simulink model "sistema_fisico"  (R2019a)
settings: Solver=VariableStepAuto  StartTime=0.0  StopTime=10.0  RelTol=1e-3
values from neighbouring files (symbols this model uses):
  b_cx = 1.0e6    (= 1000000)    [parametros.m]
  b_cy = 1.0e7    (= 10000000)    [parametros.m]
  b_h_eq = 2 * ( b_hd + i_h^2*b_hm ) / (r_hd^2)    (= 31004.4444444)    [parametros.m]
  b_hb = 1.0e8    (= 100000000)    [parametros.m]
  b_hEb = 2.2e9    (= 2200000000)    [parametros.m]
  b_t = 90.0    (= 90)    [parametros.m]
  b_tb = 5.0e6    (= 5000000)    [parametros.m]
  b_td_eq = ( b_td + i_t^2*b_tm ) / (r_td^2)    (= 21607.2)    [parametros.m]
  b_tw = 3.0e3    (= 3000)    [parametros.m]
  b_wu = 150    [parametros.m]
  g = Simulink.Parameter(9.80665)    [parametros.m]
  H_c = Simulink.Parameter(2.59)    [parametros.m]
  i_h = 22.0    (= 22)    [parametros.m]
  i_t = 30.0    (= 30)    [parametros.m]
  K_cy = 1.8e9    (= 1800000000)    [parametros.m]
  K_tw = 4.8e5    (= 480000)    [parametros.m]
  k_wu = 2.36e8    (= 236000000)    [parametros.m]
  l_h0 = Y_t0 - y_h0    [parametros.m]
  M_c_max = 50000    [parametros.m]
  M_c_min = 2000    [parametros.m]
  m_h_eq = 2 * ( J_hd_hEb + i_h^2*J_hm_hb ) / (r_hd^2)    (= 65137.7777778)    [parametros.m]
  M_s = 15000    [parametros.m]
  M_t = Simulink.Parameter(30000)    [parametros.m]
  m_td_eq = ( J_td + i_t^2*J_tm_tb ) / (r_td^2)    (= 30000)    [parametros.m]
  overload = false    [parametros.m]
  r_hd = 0.75    [parametros.m]
  r_td = 0.50    (= 0.5)    [parametros.m]
  T_hb_max = 5.0e4    (= 50000)    [parametros.m]
  T_hEb_max = 1.1e6    (= 1100000)    [parametros.m]
  T_tb_max = 5.0e3    (= 5000)    [parametros.m]
  v_h_max = 3.0    (= 3)    [parametros.m]
  x_l0 = x_t0    [parametros.m]
  x_t0 = W_c.Value / 2    [parametros.m]
  x_t_max_emer = x_t_max_oper.Value + 1.0    [parametros.m]
  x_t_max_oper = Simulink.Parameter(50.0)    [parametros.m]
  x_t_min_emer = x_t_min_oper.Value - 1.0    [parametros.m]
  x_t_min_oper = Simulink.Parameter(-30.0)    [parametros.m]
  x_td0 = x_t0    [parametros.m]
  y_h_max_emer = y_h_max_oper.Value + 1.0    [parametros.m]
  y_h_max_oper = Simulink.Parameter(40.0)    [parametros.m]
  y_h_min_emer = y_h_min_oper.Value - 1.0    [parametros.m]
  y_h_min_oper = Simulink.Parameter(-20.0)    [parametros.m]
  y_l0 = y_h0    [parametros.m]
  Y_t0 = 45.0    (= 45)    [parametros.m]
libraries: simulink x10
settings Model: Creator=Facundo  LastModifiedBy=Facundo

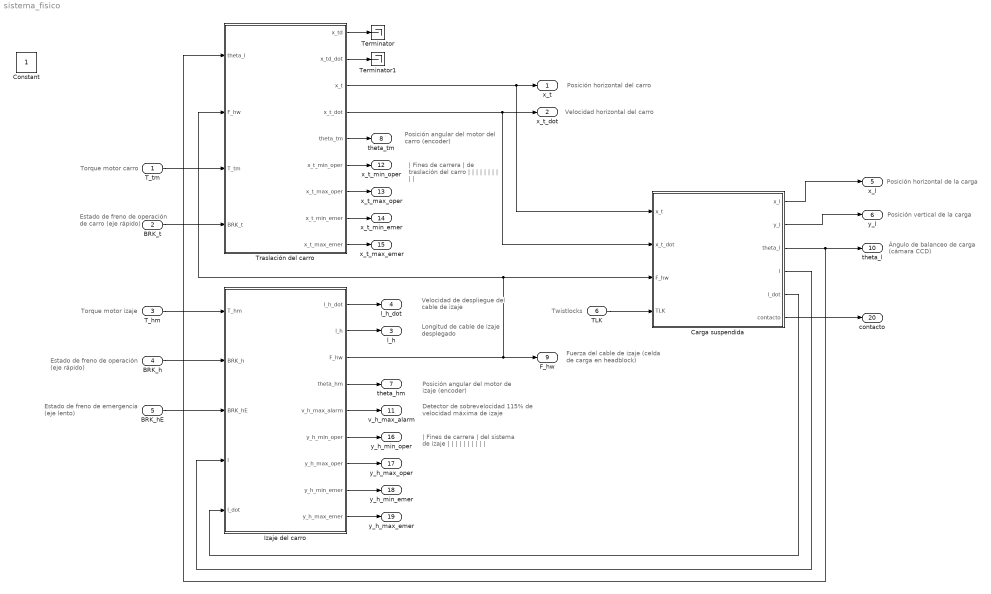
== system sistema_fisico ==
  note: Posición horizontal del carro
  note: Velocidad de despliegue
      | del cable de izaje
  note: Torque motor izaje
  note: Longitud de cable
      | de izaje desplegado
  note: Twistlocks
  note: Posición horizontal de la carga
  note: Fuerza del cable de izaje
      | (celda de carga en headblock)
  note: Detector de sobrevelocidad
      | 115% de velocidad máxima de izaje
  note: Estado de freno de emergencia
      | (eje lento)
  note: Torque motor carro
  note: Estado de freno de operación
      | (eje rápido)
  note: Posición angular del
      | motor de izaje (encoder)
  note: Posición angular del
      | motor del carro (encoder)
  note: | Fines de carrera
      | | de traslación del carro
      | |
      | |
      | |
      | |
      | |
      | |
      | |
      | |
      | |
      | |
  note: | Fines de carrera
      | | del sistema de izaje
      | |
      | |
      | |
      | |
      | |
      | |
      | |
      | |
      | |
      | |
  note: Ángulo de balanceo de carga
      | (cámara CCD)
  note: Estado de freno de
      | operación de carro
      | (eje rápido)
  note: Posición vertical de la carga
  note: Velocidad horizontal del carro
  T_tm : Inport
  BRK_t : Inport  Port=2
  T_hm : Inport  Port=3
  BRK_h : Inport  Port=4
  BRK_hE : Inport  Port=5
  TLK : Inport  Port=6  OutDataTypeStr=boolean  PortDimensions=1  SampleTime=0
  Carga suspendida : Subsystem
  Izaje del carro : Subsystem
  Terminator : Terminator
  Terminator1 : Terminator
  Traslación del carro : Subsystem
  x_t : Outport
  x_t_dot : Outport  Port=2
  l_h : Outport  Port=3
  l_h_dot : Outport  Port=4
  x_l : Outport  Port=5
  y_l : Outport  Port=6
  theta_hm : Outport  Port=7
  theta_tm : Outport  Port=8
  F_hw : Outport  Port=9
  theta_l : Outport  Port=10
  v_h_max_alarm : Outport  Port=11
  x_t_min_oper : Outport  Port=12
  x_t_max_oper : Outport  Port=13
  x_t_min_emer : Outport  Port=14
  x_t_max_emer : Outport  Port=15
  y_h_min_oper : Outport  Port=16
  y_h_max_oper : Outport  Port=17
  y_h_min_emer : Outport  Port=18
  y_h_max_emer : Outport  Port=19
  contacto : Outport  Port=20
  Constant : Constant  IOType=siggen
  wires:
  Traslación del carro/8(x_t_min_emer) -> x_t_min_emer/1
  BRK_hE/1 -> Izaje del carro/3(BRK_hE)
  Carga suspendida/2(y_l) -> y_l/1
  Izaje del carro/9(y_h_max_emer) -> y_h_max_emer/1
  Carga suspendida/3(theta_l) -> theta_l/1, Traslación del carro/1(theta_l)
  T_hm/1 -> Izaje del carro/1(T_hm)
  Izaje del carro/6(y_h_min_oper) -> y_h_min_oper/1
  Carga suspendida/1(x_l) -> x_l/1
  Izaje del carro/5(v_h_max_alarm) -> v_h_max_alarm/1
  T_tm/1 -> Traslación del carro/3(T_tm)
  Traslación del carro/4(x_t_dot) -> Carga suspendida/2(x_t_dot), x_t_dot/1
  Izaje del carro/4(theta_hm) -> theta_hm/1
  Traslación del carro/2(x_td_dot) -> Terminator1/1
  Carga suspendida/5(l_dot) -> Izaje del carro/5(l_dot)
  Izaje del carro/1(l_h_dot) -> l_h_dot/1
  Traslación del carro/5(theta_tm) -> theta_tm/1
  Izaje del carro/7(y_h_max_oper) -> y_h_max_oper/1
  Izaje del carro/2(l_h) -> l_h/1
  Izaje del carro/3(F_hw) -> F_hw/1, Carga suspendida/3(F_hw), Traslación del carro/2(F_hw)
  TLK/1 -> Carga suspendida/4(TLK)
  Traslación del carro/9(x_t_max_emer) -> x_t_max_emer/1
  Traslación del carro/1(x_td) -> Terminator/1
  Carga suspendida/6(contacto) -> contacto/1
  BRK_t/1 -> Traslación del carro/4(BRK_t)
  Traslación del carro/3(x_t) -> Carga suspendida/1(x_t), x_t/1
  Traslación del carro/6(x_t_min_oper) -> x_t_min_oper/1
  BRK_h/1 -> Izaje del carro/2(BRK_h)
  Traslación del carro/7(x_t_max_oper) -> x_t_max_oper/1
  Izaje del carro/8(y_h_min_emer) -> y_h_min_emer/1
  Carga suspendida/4(l) -> Izaje del carro/4(l)

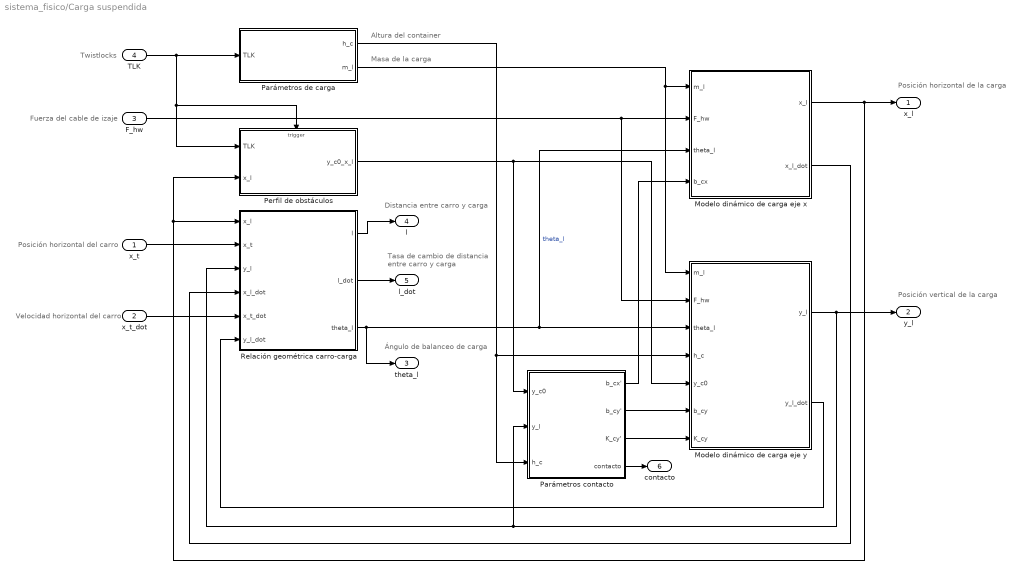
== system sistema_fisico/Carga suspendida ==
  note: Twistlocks
  note: Altura del container
  note: Posición horizontal del carro
  note: Posición vertical de la carga
  note: Velocidad horizontal del carro
  note: Distancia entre carro y carga
  note: Fuerza del cable de izaje
  note: Ángulo de balanceo de carga
  note: Tasa de cambio de distancia
      | entre carro y carga
  note: Masa de la carga
  note: Posición horizontal de la carga
  x_t : Inport  OutDataTypeStr=double  PortDimensions=1  SampleTime=0
  x_t_dot : Inport  Port=2  OutDataTypeStr=double  PortDimensions=1  SampleTime=0
  F_hw : Inport  Port=3  OutDataTypeStr=double  PortDimensions=1  SampleTime=0
  TLK : Inport  Port=4  OutDataTypeStr=boolean  PortDimensions=1  SampleTime=0
  Modelo dinámico de carga eje x : Subsystem
  Modelo dinámico de carga eje y : Subsystem
  Parámetros contacto : Subsystem
  Parámetros de carga : Subsystem
  Perfil de obstáculos : Subsystem
  Relación geométrica carro-carga : Subsystem
  x_l : Outport  OutDataTypeStr=double  PortDimensions=1  SampleTime=0
  y_l : Outport  Port=2  OutDataTypeStr=double  PortDimensions=1  SampleTime=0
  theta_l : Outport  Port=3  OutDataTypeStr=double  PortDimensions=1  SampleTime=0
  l : Outport  Port=4  OutDataTypeStr=double  PortDimensions=1  SampleTime=0
  l_dot : Outport  Port=5  OutDataTypeStr=double  PortDimensions=1  SampleTime=0
  contacto : Outport  Port=6  OutDataTypeStr=boolean  PortDimensions=1  SampleTime=0
  wires:
  Parámetros de carga/2(m_l) -> Modelo dinámico de carga eje y/1(m_l), Modelo dinámico de carga eje x/1(m_l)
  F_hw/1 -> Modelo dinámico de carga eje y/2(F_hw), Modelo dinámico de carga eje x/2(F_hw)
  Relación geométrica carro-carga/2(l_dot) -> l_dot/1
  x_t_dot/1 -> Relación geométrica carro-carga/5(x_t_dot)
  Modelo dinámico de carga eje y/1(y_l) -> y_l/1, Parámetros contacto/2(y_l), Relación geométrica carro-carga/3(y_l)
  Modelo dinámico de carga eje x/2(x_l_dot) -> Relación geométrica carro-carga/4(x_l_dot)
  Modelo dinámico de carga eje y/2(y_l_dot) -> Relación geométrica carro-carga/6(y_l_dot)
  x_t/1 -> Relación geométrica carro-carga/2(x_t)
  Modelo dinámico de carga eje x/1(x_l) -> Perfil de obstáculos/2(x_l), Relación geométrica carro-carga/1(x_l), x_l/1
  Relación geométrica carro-carga/3(theta_l) -> theta_l/1, Modelo dinámico de carga eje x/3(theta_l), Modelo dinámico de carga eje y/3(theta_l)  "theta_l"
  Parámetros contacto/1(b_cx') -> Modelo dinámico de carga eje x/4(b_cx)
  Parámetros contacto/2(b_cy') -> Modelo dinámico de carga eje y/6(b_cy)
  Parámetros contacto/3(K_cy') -> Modelo dinámico de carga eje y/7(K_cy)
  Relación geométrica carro-carga/1(l) -> l/1
  Parámetros contacto/4(contacto) -> contacto/1
  Parámetros de carga/1(h_c) -> Modelo dinámico de carga eje y/4(h_c), Parámetros contacto/3(h_c)
  Perfil de obstáculos/1(y_c0_x_l) -> Parámetros contacto/1(y_c0), Modelo dinámico de carga eje y/5(y_c0)
  TLK/1 -> Parámetros de carga/1(TLK), Perfil de obstáculos/Trigger, Perfil de obstáculos/1(TLK)

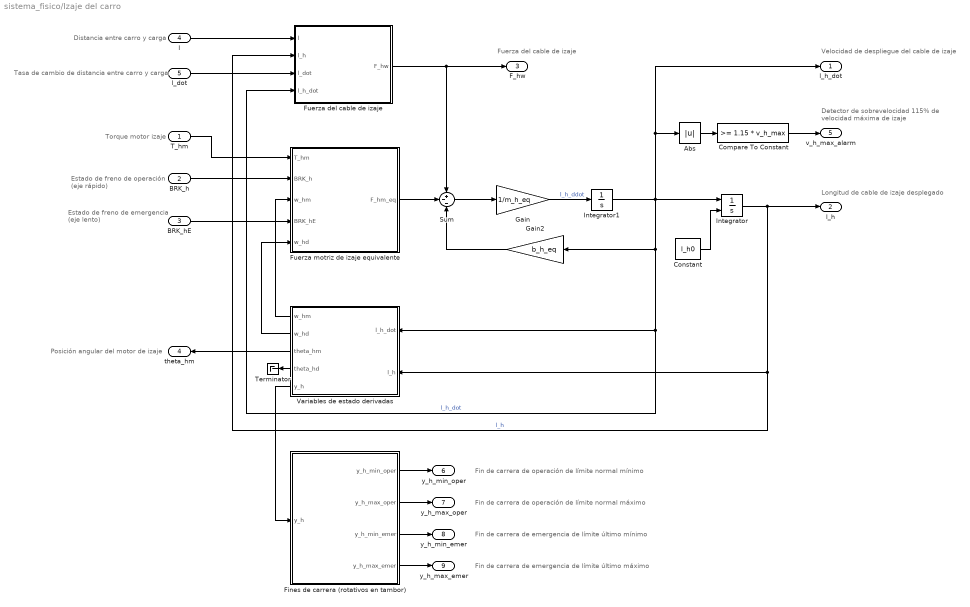
== system sistema_fisico/Izaje del carro ==
  note: Detector de sobrevelocidad
      | 115% de velocidad máxima de izaje
  note: Posición angular del motor de izaje
  note: Longitud de cable de izaje desplegado
  note: Velocidad de despliegue del cable de izaje
  note: Torque motor izaje
  note: Estado de freno de emergencia
      | (eje lento)
  note: Tasa de cambio de distancia entre carro y carga
  note: Estado de freno de operación
      | (eje rápido)
  note: Distancia entre carro y carga
  note: Fuerza del cable de izaje
  note: Fin de carrera de operación de límite normal mínimo
  note: Fin de carrera de emergencia de límite último máximo
  note: Fin de carrera de emergencia de límite último mínimo
  note: Fin de carrera de operación de límite normal máximo
  T_hm : Inport
  BRK_h : Inport  Port=2
  BRK_hE : Inport  Port=3
  l : Inport  Port=4
  l_dot : Inport  Port=5
  Abs : Abs
  Compare To Constant : simulink/Logic and Bit Operations/Compare To Constant  relop=>=  const=1.15 * v_h_max  OutDataTypeStr=boolean
  Constant : Constant  Value=l_h0
  Fines de carrera (rotativos en tambor) : Subsystem
  Fuerza del cable de izaje : Subsystem
  Fuerza motriz de izaje equivalente : Subsystem
  Gain : Gain  Gain=1/m_h_eq
  Gain2 : Gain  Gain=b_h_eq
  Integrator : Integrator  InitialConditionSource=external
  Integrator1 : Integrator
  Sum : Sum  Inputs=+--
  Terminator : Terminator
  Variables de estado derivadas : Subsystem
  l_h_dot : Outport
  l_h : Outport  Port=2
  F_hw : Outport  Port=3
  theta_hm : Outport  Port=4
  v_h_max_alarm : Outport  Port=5
  y_h_min_oper : Outport  Port=6  OutDataTypeStr=boolean  PortDimensions=1  SampleTime=0
  y_h_max_oper : Outport  Port=7  OutDataTypeStr=boolean  PortDimensions=1  SampleTime=0
  y_h_min_emer : Outport  Port=8  OutDataTypeStr=boolean  PortDimensions=1  SampleTime=0
  y_h_max_emer : Outport  Port=9  OutDataTypeStr=boolean  PortDimensions=1  SampleTime=0
  wires:
  Integrator/1 -> l_h/1, Fuerza del cable de izaje/2(l_h), Variables de estado derivadas/2(l_h)  "l_h"
  Integrator1/1 -> l_h_dot/1, Abs/1, Fuerza del cable de izaje/4(l_h_dot), Variables de estado derivadas/1(l_h_dot), Gain2/1, Integrator/1  "l_h_dot"
  T_hm/1 -> Fuerza motriz de izaje equivalente/1(T_hm)
  l/1 -> Fuerza del cable de izaje/1(l)
  l_dot/1 -> Fuerza del cable de izaje/3(l_dot)
  Fuerza del cable de izaje/1(F_hw) -> F_hw/1, Sum/1
  Gain2/1 -> Sum/3
  Fuerza motriz de izaje equivalente/1(F_hm_eq) -> Sum/2
  Variables de estado derivadas/1(w_hm) -> Fuerza motriz de izaje equivalente/3(w_hm)
  Sum/1 -> Gain/1
  Variables de estado derivadas/2(w_hd) -> Fuerza motriz de izaje equivalente/5(w_hd)
  BRK_h/1 -> Fuerza motriz de izaje equivalente/2(BRK_h)
  BRK_hE/1 -> Fuerza motriz de izaje equivalente/4(BRK_hE)
  Gain/1 -> Integrator1/1  "l_h_ddot"
  Constant/1 -> Integrator/2
  Variables de estado derivadas/3(theta_hm) -> theta_hm/1
  Abs/1 -> Compare To Constant/1
  Compare To Constant/1 -> v_h_max_alarm/1
  Fines de carrera (rotativos en tambor)/1(y_h_min_oper) -> y_h_min_oper/1
  Fines de carrera (rotativos en tambor)/4(y_h_max_emer) -> y_h_max_emer/1
  Fines de carrera (rotativos en tambor)/3(y_h_min_emer) -> y_h_min_emer/1
  Fines de carrera (rotativos en tambor)/2(y_h_max_oper) -> y_h_max_oper/1
  Variables de estado derivadas/5(y_h) -> Fines de carrera (rotativos en tambor)/1(y_h)
  Variables de estado derivadas/4(theta_hd) -> Terminator/1

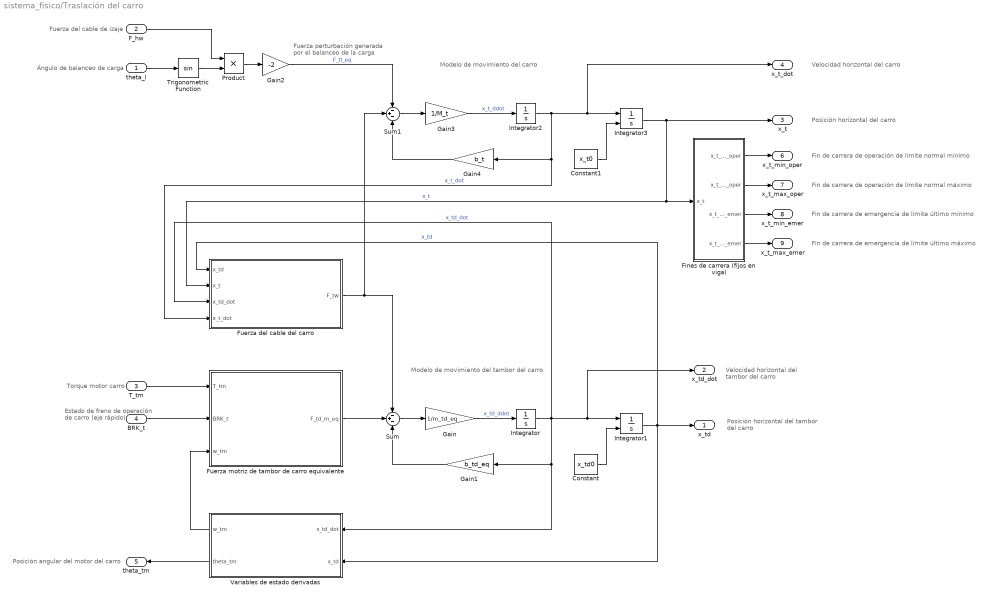
== system sistema_fisico/Traslación del carro ==
  note: Posición angular del motor del carro
  note: Velocidad horizontal
      | del tambor del carro
  note: Modelo de movimiento del tambor del carro
  note: Modelo de movimiento del carro
  note: Velocidad horizontal del carro
  note: Estado de freno de
      | operación de carro
      | (eje rápido)
  note: Fuerza del cable de izaje
  note: Fuerza perturbación generada
      | por el balanceo de la carga
  note: Posición horizontal del carro
  note: Torque motor carro
  note: Ángulo de balanceo de carga
  note: Posición horizontal
      | del tambor del carro
  note: Fin de carrera de operación de límite normal mínimo
  note: Fin de carrera de operación de límite normal máximo
  note: Fin de carrera de emergencia de límite último mínimo
  note: Fin de carrera de emergencia de límite último máximo
  theta_l : Inport  OutDataTypeStr=double  PortDimensions=1  SampleTime=0
  F_hw : Inport  Port=2  OutDataTypeStr=double  PortDimensions=1  SampleTime=0
  T_tm : Inport  Port=3
  BRK_t : Inport  Port=4
  Constant : Constant  Value=x_td0
  Constant1 : Constant  Value=x_t0
  Fines de carrera (fijos en viga) : Subsystem
  Fuerza del cable del carro : Subsystem
  Fuerza motriz de tambor de carro equivalente : Subsystem
  Gain : Gain  Gain=1/m_td_eq
  Gain1 : Gain  Gain=b_td_eq
  Gain2 : Gain  Gain=-2
  Gain3 : Gain  Gain=1/M_t
  Gain4 : Gain  Gain=b_t
  Integrator : Integrator
  Integrator1 : Integrator  InitialConditionSource=external
  Integrator2 : Integrator
  Integrator3 : Integrator  InitialConditionSource=external
  Product : Product
  Sum : Sum  Inputs=-+-
  Sum1 : Sum  Inputs=-+-
  Trigonometric Function : Trigonometry
  Variables de estado derivadas : Subsystem
  x_td : Outport  OutDataTypeStr=double  PortDimensions=1  SampleTime=0
  x_td_dot : Outport  Port=2  OutDataTypeStr=double  PortDimensions=1  SampleTime=0
  x_t : Outport  Port=3  OutDataTypeStr=double  PortDimensions=1  SampleTime=0
  x_t_dot : Outport  Port=4  OutDataTypeStr=double  PortDimensions=1  SampleTime=0
  theta_tm : Outport  Port=5  OutDataTypeStr=double  PortDimensions=1  SampleTime=0
  x_t_min_oper : Outport  Port=6  OutDataTypeStr=boolean  PortDimensions=1  SampleTime=0
  x_t_max_oper : Outport  Port=7  OutDataTypeStr=boolean  PortDimensions=1  SampleTime=0
  x_t_min_emer : Outport  Port=8  OutDataTypeStr=boolean  PortDimensions=1  SampleTime=0
  x_t_max_emer : Outport  Port=9  OutDataTypeStr=boolean  PortDimensions=1  SampleTime=0
  wires:
  Integrator1/1 -> Variables de estado derivadas/2(x_td), Fuerza del cable del carro/1(x_td), x_td/1  "x_td"
  Gain3/1 -> Integrator2/1  "x_t_ddot"
  Fuerza del cable del carro/1(F_tw) -> Sum1/2, Sum/1
  Sum/1 -> Gain/1
  Integrator/1 -> Fuerza del cable del carro/3(x_td_dot), Variables de estado derivadas/1(x_td_dot), Gain1/1, x_td_dot/1, Integrator1/1  "x_td_dot"
  F_hw/1 -> Product/1
  Fuerza motriz de tambor de carro equivalente/1(F_td_m_eq) -> Sum/2
  Constant/1 -> Integrator1/2
  Gain1/1 -> Sum/3
  Integrator2/1 -> Fuerza del cable del carro/4(x_t_dot), Gain4/1, x_t_dot/1, Integrator3/1  "x_t_dot"
  Sum1/1 -> Gain3/1
  theta_l/1 -> Trigonometric Function/1
  Gain4/1 -> Sum1/3
  Integrator3/1 -> x_t/1, Fuerza del cable del carro/2(x_t), Fines de carrera (fijos en viga)/1(x_t)  "x_t"
  Gain2/1 -> Sum1/1  "F_tl_eq"
  T_tm/1 -> Fuerza motriz de tambor de carro equivalente/1(T_tm)
  BRK_t/1 -> Fuerza motriz de tambor de carro equivalente/2(BRK_t)
  Variables de estado derivadas/1(w_tm) -> Fuerza motriz de tambor de carro equivalente/3(w_tm)
  Constant1/1 -> Integrator3/2
  Trigonometric Function/1 -> Product/2
  Product/1 -> Gain2/1
  Gain/1 -> Integrator/1  "x_td_ddot"
  Variables de estado derivadas/2(theta_tm) -> theta_tm/1
  Fines de carrera (fijos en viga)/1(x_t_min_oper) -> x_t_min_oper/1
  Fines de carrera (fijos en viga)/2(x_t_max_oper) -> x_t_max_oper/1
  Fines de carrera (fijos en viga)/3(x_t_min_emer) -> x_t_min_emer/1
  Fines de carrera (fijos en viga)/4(x_t_max_emer) -> x_t_max_emer/1

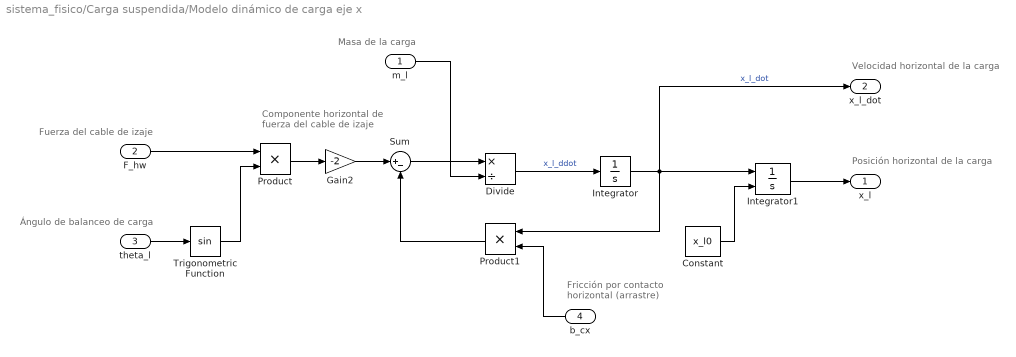
== system sistema_fisico/Carga suspendida/Modelo dinámico de carga eje x ==
  note: Componente horizontal de
      | fuerza del cable de izaje
  note: Posición horizontal de la carga
  note: Velocidad horizontal de la carga
  note: Fuerza del cable de izaje
  note: Masa de la carga
  note: Fricción por contacto
      | horizontal (arrastre)
  note: Ángulo de balanceo de carga
  m_l : Inport  OutDataTypeStr=double  PortDimensions=1  SampleTime=0
  F_hw : Inport  Port=2  OutDataTypeStr=double  PortDimensions=1  SampleTime=0
  theta_l : Inport  Port=3  OutDataTypeStr=double  PortDimensions=1  SampleTime=0
  b_cx : Inport  Port=4  OutDataTypeStr=double  PortDimensions=1  SampleTime=0
  Constant : Constant  Value=x_l0
  Divide : Product  Inputs=*/
  Gain2 : Gain  Gain=-2
  Integrator : Integrator
  Integrator1 : Integrator  InitialConditionSource=external
  Product : Product
  Product1 : Product
  Sum : Sum  Inputs=|+-
  Trigonometric Function : Trigonometry
  x_l : Outport  OutDataTypeStr=double  PortDimensions=1  SampleTime=0
  x_l_dot : Outport  Port=2  OutDataTypeStr=double  PortDimensions=1  SampleTime=0
  wires:
  F_hw/1 -> Product/1
  Product1/1 -> Sum/2
  theta_l/1 -> Trigonometric Function/1
  b_cx/1 -> Product1/2
  Sum/1 -> Divide/1
  Integrator/1 -> x_l_dot/1, Integrator1/1, Product1/1  "x_l_dot"
  Product/1 -> Gain2/1
  Divide/1 -> Integrator/1  "x_l_ddot"
  Constant/1 -> Integrator1/2
  Integrator1/1 -> x_l/1
  Gain2/1 -> Sum/1
  m_l/1 -> Divide/2
  Trigonometric Function/1 -> Product/2

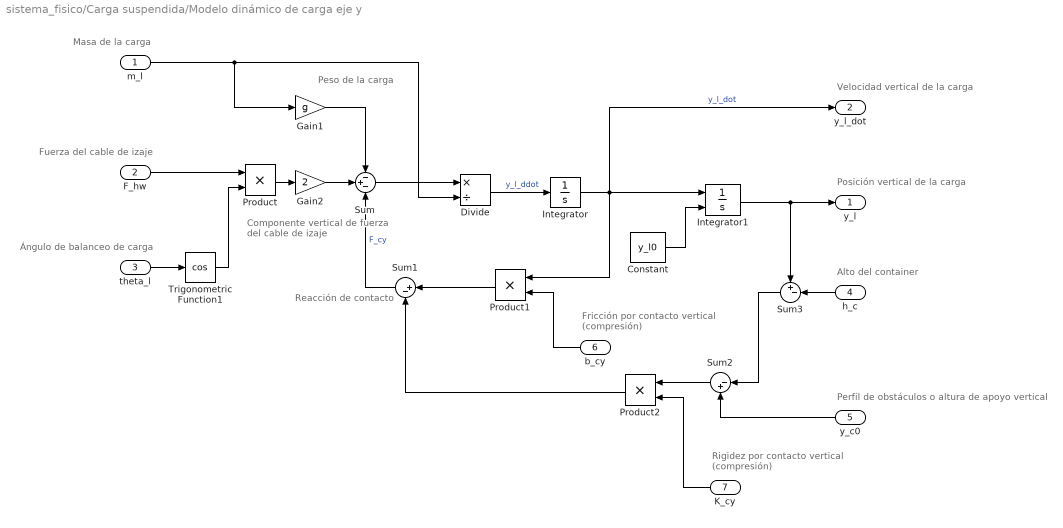
== system sistema_fisico/Carga suspendida/Modelo dinámico de carga eje y ==
  note: Reacción de contacto
  note: Peso de la carga
  note: Componente vertical de
      | fuerza del cable de izaje
  note: Posición vertical de la carga
  note: Velocidad vertical de la carga
  note: Fricción por contacto
      | vertical (compresión)
  note: Rigidez por contacto
      | vertical (compresión)
  note: Masa de la carga
  note: Fuerza del cable de izaje
  note: Perfil de obstáculos o altura de apoyo vertical
  note: Alto del container
  note: Ángulo de balanceo de carga
  m_l : Inport  OutDataTypeStr=double  PortDimensions=1  SampleTime=0
  F_hw : Inport  Port=2  OutDataTypeStr=double  PortDimensions=1  SampleTime=0
  theta_l : Inport  Port=3  OutDataTypeStr=double  PortDimensions=1  SampleTime=0
  h_c : Inport  Port=4  OutDataTypeStr=double  PortDimensions=1  SampleTime=0
  y_c0 : Inport  Port=5  OutDataTypeStr=double  PortDimensions=1  SampleTime=0
  b_cy : Inport  Port=6  OutDataTypeStr=double  PortDimensions=1  SampleTime=0
  K_cy : Inport  Port=7  OutDataTypeStr=double  PortDimensions=1  SampleTime=0
  Constant : Constant  Value=y_l0
  Divide : Product  Inputs=*/
  Gain1 : Gain  Gain=g
  Gain2 : Gain  Gain=2
  Integrator : Integrator
  Integrator1 : Integrator  InitialConditionSource=external
  Product : Product
  Product1 : Product
  Product2 : Product
  Sum : Sum  Inputs=-+-
  Sum1 : Sum  Inputs=|+-
  Sum2 : Sum  Inputs=|-+
  Sum3 : Sum  Inputs=+-|
  Trigonometric Function1 : Trigonometry  Operator=cos
  y_l : Outport  OutDataTypeStr=double  PortDimensions=1  SampleTime=0
  y_l_dot : Outport  Port=2  OutDataTypeStr=double  PortDimensions=1  SampleTime=0
  wires:
  F_hw/1 -> Product/1
  theta_l/1 -> Trigonometric Function1/1
  b_cy/1 -> Product1/2
  Integrator/1 -> y_l_dot/1, Integrator1/1, Product1/1  "y_l_dot"
  Divide/1 -> Integrator/1  "y_l_ddot"
  Constant/1 -> Integrator1/2
  Integrator1/1 -> y_l/1, Sum3/1
  Product/1 -> Gain2/1
  Product1/1 -> Sum1/1
  Sum1/1 -> Sum/3  "F_cy"
  Gain1/1 -> Sum/1
  y_c0/1 -> Sum2/2
  Sum2/1 -> Product2/1
  K_cy/1 -> Product2/2
  Product2/1 -> Sum1/2
  Gain2/1 -> Sum/2
  Sum/1 -> Divide/1
  m_l/1 -> Gain1/1, Divide/2
  h_c/1 -> Sum3/2
  Sum3/1 -> Sum2/1
  Trigonometric Function1/1 -> Product/2

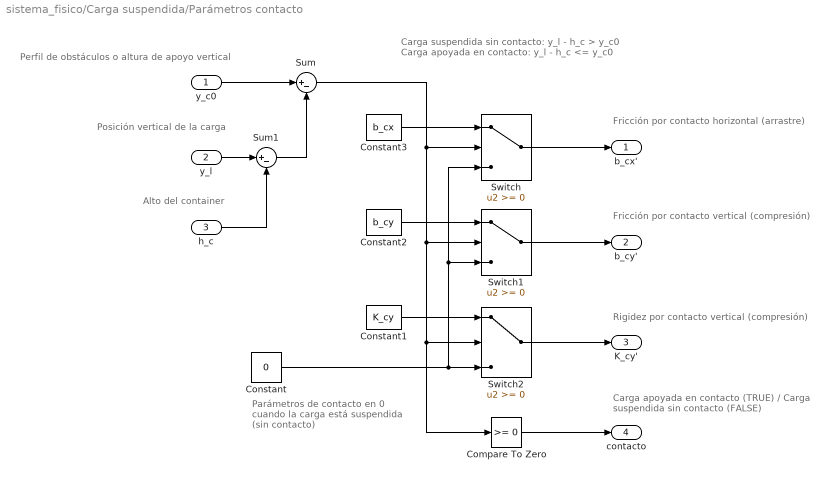
== system sistema_fisico/Carga suspendida/Parámetros contacto ==
  note: Fricción por contacto horizontal (arrastre)
  note: Fricción por contacto vertical (compresión)
  note: Rigidez por contacto vertical (compresión)
  note: Perfil de obstáculos o altura de apoyo vertical
  note: Posición vertical de la carga
  note: Alto del container
  note: Parámetros de contacto en 0
      | cuando la carga está suspendida
      | (sin contacto)
  note: Carga suspendida sin contacto: y_l - h_c > y_c0
      | Carga apoyada en contacto: y_l - h_c <= y_c0
  note: Carga apoyada en contacto (TRUE) /
      | Carga suspendida sin contacto (FALSE)
  y_c0 : Inport  OutDataTypeStr=double  PortDimensions=1  SampleTime=0
  y_l : Inport  Port=2  OutDataTypeStr=double  PortDimensions=1  SampleTime=0
  h_c : Inport  Port=3  OutDataTypeStr=double  PortDimensions=1  SampleTime=0
  Compare To Zero : simulink/Logic and Bit Operations/Compare To Zero  relop=>=  OutDataTypeStr=boolean
  Constant : Constant  Value=0
  Constant1 : Constant  Value=K_cy
  Constant2 : Constant  Value=b_cy
  Constant3 : Constant  Value=b_cx
  Sum : Sum  Inputs=|+-
  Sum1 : Sum  Inputs=|+-
  Switch : Switch
  Switch1 : Switch
  Switch2 : Switch
  b_cx' : Outport  OutDataTypeStr=double  PortDimensions=1  SampleTime=0
  b_cy' : Outport  Port=2  OutDataTypeStr=double  PortDimensions=1  SampleTime=0
  K_cy' : Outport  Port=3  OutDataTypeStr=double  PortDimensions=1  SampleTime=0
  contacto : Outport  Port=4  OutDataTypeStr=boolean  PortDimensions=1  SampleTime=0
  wires:
  y_c0/1 -> Sum/1
  Constant2/1 -> Switch1/1
  Constant1/1 -> Switch2/1
  Switch/1 -> b_cx'/1
  Sum/1 -> Switch1/2, Compare To Zero/1, Switch2/2, Switch/2
  Switch2/1 -> K_cy'/1
  Switch1/1 -> b_cy'/1
  Constant/1 -> Switch/3, Switch1/3, Switch2/3
  Constant3/1 -> Switch/1
  Sum1/1 -> Sum/2
  y_l/1 -> Sum1/1
  h_c/1 -> Sum1/2
  Compare To Zero/1 -> contacto/1

== system sistema_fisico/Carga suspendida/Parámetros de carga ==
  note: Twistlocks
  note: Masa de la carga total
  note: Alto del container
      | (afecta altura inferior)
  note: Masa del spreader
  note: Masa del contenedor
      | y carga
  TLK : Inport  OutDataTypeStr=boolean  PortDimensions=1  SampleTime=0
  "Generate random load " : Subsystem  TreatAsAtomicUnit=on
  Sum : Sum  Inputs=++|
  Switch : Switch  Criteria=u2 ~= 0
  Switch1 : Switch  Criteria=u2 ~= 0
  h_c1 : Constant  Value=H_c
  h_c2 : Constant  Value=0
  h_c3 : Constant  Value=M_s
  h_c4 : Constant  Value=0
  h_c : Outport
  m_l : Outport  Port=2
  wires:
  TLK/1 -> "Generate random load "/Trigger, Switch1/2, Switch/2
  Switch/1 -> h_c/1
  Sum/1 -> m_l/1
  Switch1/1 -> Sum/2  "M_cx"
  "Generate random load "/1(M_cx) -> Switch1/1
  h_c3/1 -> Sum/1  "M_s"
  h_c2/1 -> Switch/3
  h_c4/1 -> Switch1/3
  h_c1/1 -> Switch/1

== system sistema_fisico/Carga suspendida/Perfil de obstáculos ==
  note: Perfil de obstáculos para x_l
  note: Se actualiza el perfil de obstá culos cuando
      | se cierran (TLK ↑) o abren (TLK ↓) los twistlocks
  note: Perfil de obstáculos
  note: Guarda perfil de obstáculos en workspace
      | para posterior análisis (plot_perfil_obstaculos.m)
  TLK : Inport  PortDimensions=1
  x_l : Inport  Port=2  OutDataTypeStr=double  PortDimensions=1
  Trigger : TriggerPort  TriggerType=either  VariantControl=Variant  PortDimensions=1
  Constant : Constant  Value=H_c
  Constant1 : Constant  Value=x_t_min_oper
  Constant2 : Constant  Value=x_t_max_oper
  Constant3 : Constant  Value=y_h_min_oper
  MATLAB Function : MATLAB Function  TreatAsAtomicUnit=on
  To Workspace : ToWorkspace  VariableName=y_c0  SaveFormat=Structure With Time  SampleTime=-1
  y_c0_x_l : Outport  OutDataTypeStr=double  PortDimensions=1  InitialOutput=y_h_min_oper
  wires:
  MATLAB Function/1(y_c0_x_l) -> y_c0_x_l/1
  TLK/1 -> MATLAB Function/2(TLK)
  x_l/1 -> MATLAB Function/1(x_l)
  Constant/1 -> MATLAB Function/3(H_c)
  Constant1/1 -> MATLAB Function/4(x_t_min_oper)
  Constant2/1 -> MATLAB Function/5(x_t_max_oper)
  Constant3/1 -> MATLAB Function/6(y_h_min_oper)
  MATLAB Function/2(y_c0) -> To Workspace/1

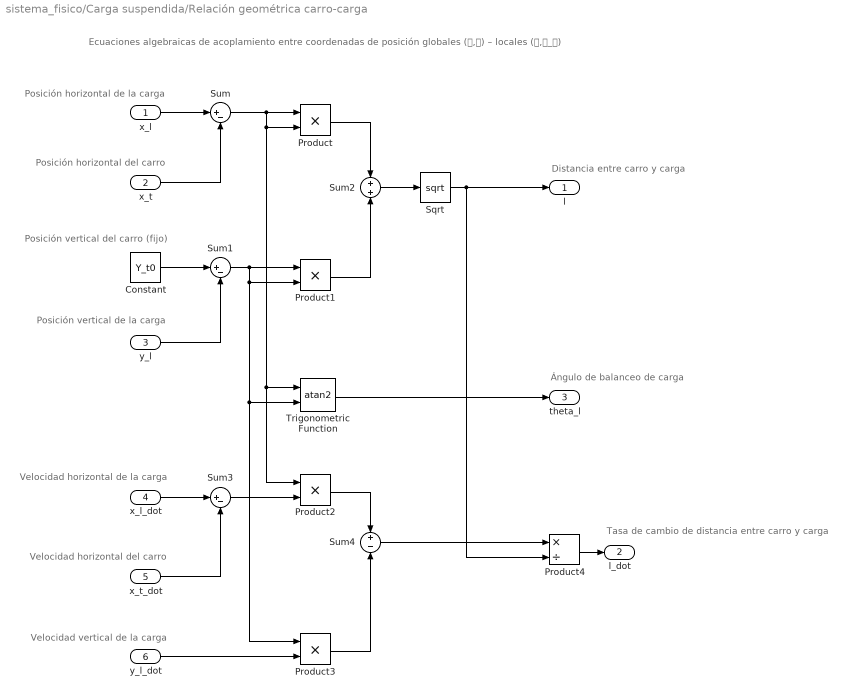
== system sistema_fisico/Carga suspendida/Relación geométrica carro-carga ==
  note: Ecuaciones algebraicas de acoplamiento entre coordenadas de posición globales (𝑥,𝑦) – locales (𝑙,𝜃_𝑙)
  note: Posición horizontal de la carga
  note: Posición horizontal del carro
  note: Posición vertical del carro (fijo)
  note: Posición vertical de la carga
  note: Distancia entre carro y carga
  note: Tasa de cambio de distancia entre carro y carga
  note: Ángulo de balanceo de carga
  note: Velocidad horizontal de la carga
  note: Velocidad horizontal del carro
  note: Velocidad vertical de la carga
  x_l : Inport
  x_t : Inport  Port=2
  y_l : Inport  Port=3
  x_l_dot : Inport  Port=4
  x_t_dot : Inport  Port=5
  y_l_dot : Inport  Port=6
  Constant : Constant  Value=Y_t0
  Product{,1..3} (4 alike) : Product
  Product4 : Product  Inputs=*/
  Sqrt : Sqrt  SaturateOnIntegerOverflow=on
  Sum : Sum  Inputs=|+-
  Sum1 : Sum  Inputs=|+-
  Sum2 : Sum  Inputs=+|+
  Sum3 : Sum  Inputs=|+-
  Sum4 : Sum  Inputs=+|-
  Trigonometric Function : Trigonometry  Operator=atan2
  l : Outport
  l_dot : Outport  Port=2
  theta_l : Outport  Port=3
  wires:
  x_t/1 -> Sum/2
  x_l/1 -> Sum/1
  Sum/1 -> Product/1, Product2/1, Trigonometric Function/1, Product/2
  Product/1 -> Sum2/1
  y_l/1 -> Sum1/2
  Sum1/1 -> Product1/1, Product3/1, Trigonometric Function/2, Product1/2
  Constant/1 -> Sum1/1
  Product1/1 -> Sum2/2
  Sum2/1 -> Sqrt/1
  Trigonometric Function/1 -> theta_l/1
  x_l_dot/1 -> Sum3/1
  x_t_dot/1 -> Sum3/2
  Sum3/1 -> Product2/2
  y_l_dot/1 -> Product3/2
  Product2/1 -> Sum4/1
  Product3/1 -> Sum4/2
  Sum4/1 -> Product4/1
  Product4/1 -> l_dot/1
  Sqrt/1 -> Product4/2, l/1

== system sistema_fisico/Izaje del carro/Fines de carrera (rotativos en tambor) ==
  note: Fines de carrera son rotativos sobre tambor (theta_hd). Por simplicidad se usa la variable equivalente lineal (y_h)
  note: Fin de carrera de operación de límite normal mínimo
  note: Fin de carrera de operación de límite normal máximo
  note: Fin de carrera de emergencia de límite último mínimo
  note: Fin de carrera de operación de límite último máximo
  note: Altura de la carga sin balanceo
  y_h : Inport
  Compare To Constant : simulink/Logic and Bit Operations/Compare To Constant  relop=<=  const=y_h_min_oper  OutDataTypeStr=boolean
  Compare To Constant1 : simulink/Logic and Bit Operations/Compare To Constant  relop=>=  const=y_h_max_oper  OutDataTypeStr=boolean
  Compare To Constant2 : simulink/Logic and Bit Operations/Compare To Constant  relop=<=  const=y_h_min_emer  OutDataTypeStr=boolean
  Compare To Constant3 : simulink/Logic and Bit Operations/Compare To Constant  relop=>=  const=y_h_max_emer  OutDataTypeStr=boolean
  y_h_min_oper : Outport  OutDataTypeStr=boolean  PortDimensions=1  SampleTime=0
  y_h_max_oper : Outport  Port=2  OutDataTypeStr=boolean  PortDimensions=1  SampleTime=0
  y_h_min_emer : Outport  Port=3  OutDataTypeStr=boolean  PortDimensions=1  SampleTime=0
  y_h_max_emer : Outport  Port=4  OutDataTypeStr=boolean  PortDimensions=1  SampleTime=0
  wires:
  Compare To Constant2/1 -> y_h_min_emer/1
  Compare To Constant/1 -> y_h_min_oper/1
  Compare To Constant1/1 -> y_h_max_oper/1
  y_h/1 -> Compare To Constant3/1, Compare To Constant2/1, Compare To Constant1/1, Compare To Constant/1
  Compare To Constant3/1 -> y_h_max_emer/1

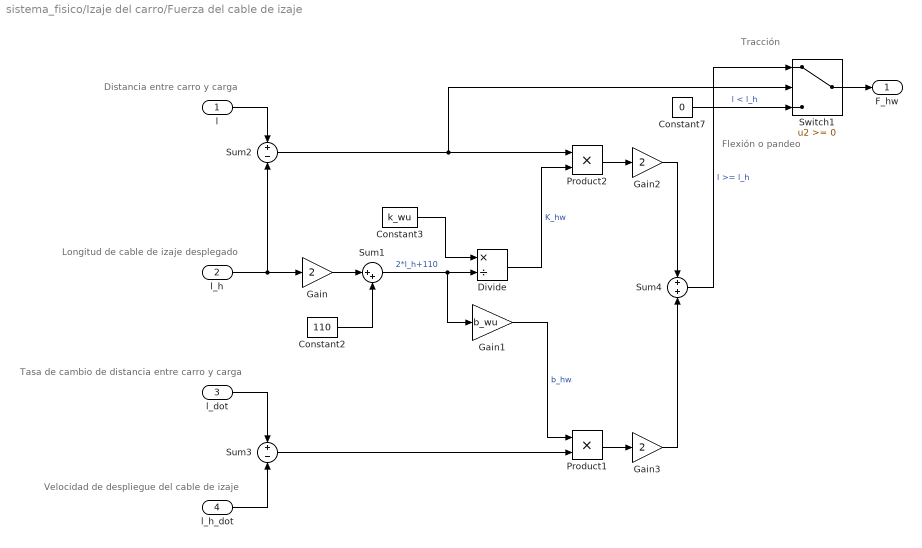
== system sistema_fisico/Izaje del carro/Fuerza del cable de izaje ==
  note: Flexión o pandeo
  note: Tracción
  note: Distancia entre carro y carga
  note: Tasa de cambio de distancia entre carro y carga
  note: Longitud de cable de izaje desplegado
  note: Velocidad de despliegue del cable de izaje
  l : Inport
  l_h : Inport  Port=2
  l_dot : Inport  Port=3
  l_h_dot : Inport  Port=4
  Constant2 : Constant  Value=110
  Constant3 : Constant  Value=k_wu
  Constant7 : Constant  Value=0
  Divide : Product  Inputs=*/
  Gain : Gain  Gain=2
  Gain1 : Gain  Gain=b_wu
  Gain2 : Gain  Gain=2
  Gain3 : Gain  Gain=2
  Product1 : Product
  Product2 : Product
  Sum1 : Sum  Inputs=|++
  Sum2 : Sum  Inputs=+-
  Sum3 : Sum  Inputs=+-
  Sum4 : Sum
  Switch1 : Switch
  F_hw : Outport
  wires:
  l_dot/1 -> Sum3/1
  Constant2/1 -> Sum1/2
  Sum1/1 -> Gain1/1, Divide/2  "2*l_h+110"
  l/1 -> Sum2/1
  Product1/1 -> Gain3/1
  Sum3/1 -> Product1/2
  l_h_dot/1 -> Sum3/2
  l_h/1 -> Gain/1, Sum2/2
  Divide/1 -> Product2/2  "K_hw"
  Sum2/1 -> Switch1/2, Product2/1
  Constant3/1 -> Divide/1
  Gain1/1 -> Product1/1  "b_hw"
  Product2/1 -> Gain2/1
  Switch1/1 -> F_hw/1
  Sum4/1 -> Switch1/1  "l >= l_h"
  Constant7/1 -> Switch1/3  "l < l_h"
  Gain/1 -> Sum1/1
  Gain2/1 -> Sum4/1
  Gain3/1 -> Sum4/2

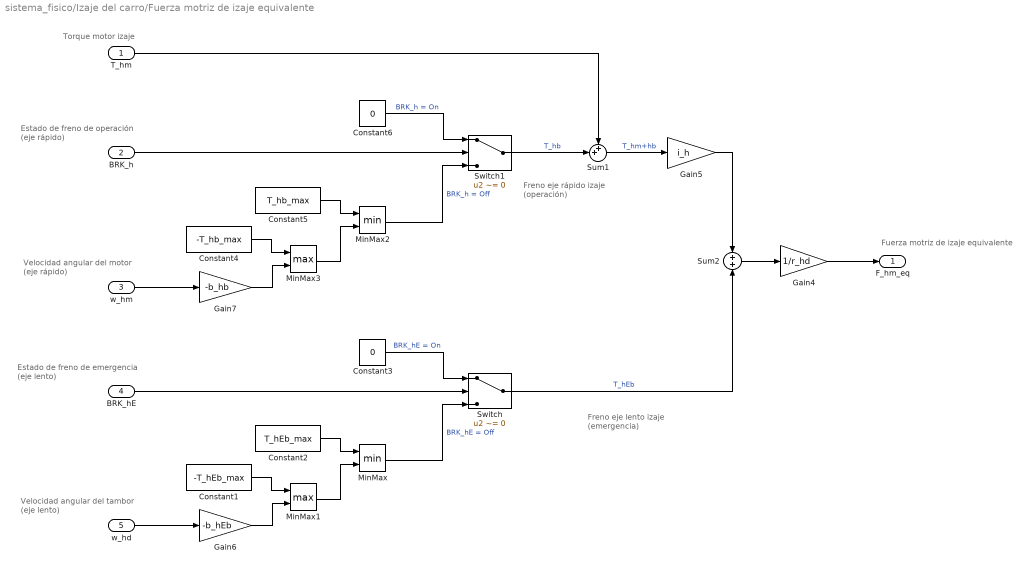
== system sistema_fisico/Izaje del carro/Fuerza motriz de izaje equivalente ==
  note: Fuerza motriz de izaje equivalente
  note: Torque motor izaje
  note: Freno eje lento izaje
      | (emergencia)
  note: Freno eje rápido izaje
      | (operación)
  note: Estado de freno de operación
      | (eje rápido)
  note: Estado de freno de emergencia
      | (eje lento)
  note: Velocidad angular del tambor
      | (eje lento)
  note: Velocidad angular del motor
      | (eje rápido)
  T_hm : Inport
  BRK_h : Inport  Port=2  OutDataTypeStr=boolean
  w_hm : Inport  Port=3
  BRK_hE : Inport  Port=4  OutDataTypeStr=boolean
  w_hd : Inport  Port=5
  Constant1 : Constant  Value=-T_hEb_max
  Constant2 : Constant  Value=T_hEb_max
  Constant3 : Constant  Value=0
  Constant4 : Constant  Value=-T_hb_max
  Constant5 : Constant  Value=T_hb_max
  Constant6 : Constant  Value=0
  Gain4 : Gain  Gain=1/r_hd
  Gain5 : Gain  Gain=i_h
  Gain6 : Gain  Gain=-b_hEb
  Gain7 : Gain  Gain=-b_hb
  MinMax : MinMax  Inputs=2
  MinMax1 : MinMax  Function=max  Inputs=2
  MinMax2 : MinMax  Inputs=2
  MinMax3 : MinMax  Function=max  Inputs=2
  Sum1 : Sum  Inputs=++|
  Sum2 : Sum  Inputs=2
  Switch : Switch  Criteria=u2 ~= 0
  Switch1 : Switch  Criteria=u2 ~= 0
  F_hm_eq : Outport
  wires:
  MinMax3/1 -> MinMax2/2
  MinMax1/1 -> MinMax/2
  Constant1/1 -> MinMax1/1
  MinMax2/1 -> Switch1/3  "BRK_h = Off"
  Gain5/1 -> Sum2/1
  Constant4/1 -> MinMax3/1
  T_hm/1 -> Sum1/1
  w_hm/1 -> Gain7/1
  Constant5/1 -> MinMax2/1
  w_hd/1 -> Gain6/1
  Gain7/1 -> MinMax3/2
  BRK_h/1 -> Switch1/2
  Constant6/1 -> Switch1/1  "BRK_h = On"
  MinMax/1 -> Switch/3  "BRK_hE = Off"
  Sum1/1 -> Gain5/1  "T_hm+hb"
  Switch1/1 -> Sum1/2  "T_hb"
  Constant3/1 -> Switch/1  "BRK_hE = On"
  BRK_hE/1 -> Switch/2
  Constant2/1 -> MinMax/1
  Gain6/1 -> MinMax1/2
  Gain4/1 -> F_hm_eq/1
  Sum2/1 -> Gain4/1
  Switch/1 -> Sum2/2  "T_hEb"

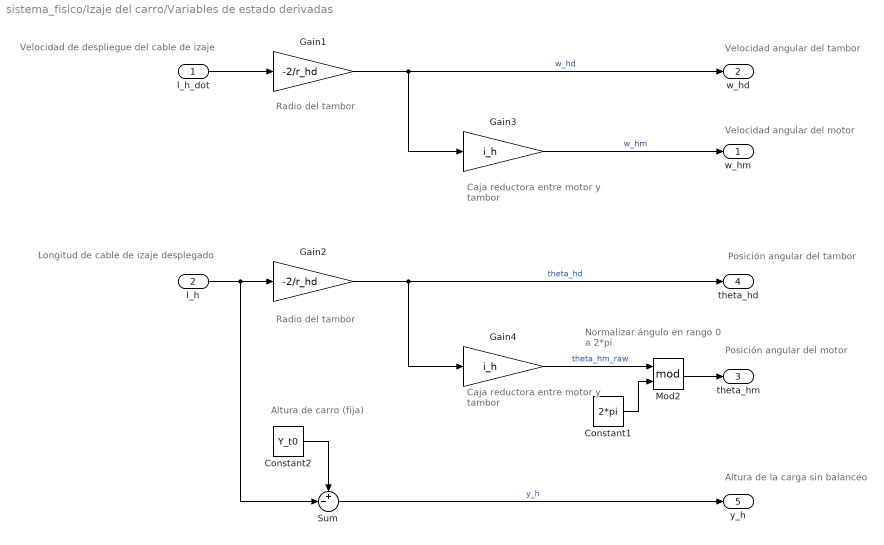
== system sistema_fisico/Izaje del carro/Variables de estado derivadas ==
  note: Velocidad angular del tambor
  note: Caja reductora
      | entre motor y tambor
  note: Velocidad angular del motor
  note: Velocidad de despliegue del cable de izaje
  note: Longitud de cable de izaje desplegado
  note: Posición angular del motor
  note: Caja reductora
      | entre motor y tambor
  note: Radio del tambor
  note: Radio del tambor
  note: Normalizar ángulo en
      | rango 0 a 2*pi
  note: Posición angular del tambor
  note: Altura de carro (fija)
  note: Altura de la carga sin balanceo
  l_h_dot : Inport
  l_h : Inport  Port=2
  Constant1 : Constant  Value=2*pi
  Constant2 : Constant  Value=Y_t0
  Gain1 : Gain  Gain=-2/r_hd
  Gain2 : Gain  Gain=-2/r_hd
  Gain3 : Gain  Gain=i_h
  Gain4 : Gain  Gain=i_h
  Mod2 : Math  Operator=mod  SaturateOnIntegerOverflow=on
  Sum : Sum  Inputs=+-|
  w_hm : Outport
  w_hd : Outport  Port=2
  theta_hm : Outport  Port=3
  theta_hd : Outport  Port=4
  y_h : Outport  Port=5
  wires:
  Gain1/1 -> w_hd/1, Gain3/1  "w_hd"
  l_h_dot/1 -> Gain1/1
  Gain3/1 -> w_hm/1  "w_hm"
  Gain2/1 -> theta_hd/1, Gain4/1  "theta_hd"
  l_h/1 -> Sum/2, Gain2/1
  Gain4/1 -> Mod2/1  "theta_hm_raw"
  Constant1/1 -> Mod2/2
  Mod2/1 -> theta_hm/1
  Constant2/1 -> Sum/1
  Sum/1 -> y_h/1  "y_h"

== system sistema_fisico/Traslación del carro/Fines de carrera (fijos en viga) ==
  note: Posición horizontal del carro
  note: Fin de carrera de operación de límite normal mínimo
  note: Fin de carrera de operación de límite normal máximo
  note: Fin de carrera de emergencia de límite último mínimo
  note: Fin de carrera de operación de límite último máximo
  x_t : Inport
  Compare To Constant : simulink/Logic and Bit Operations/Compare To Constant  relop=<=  const=x_t_min_oper  OutDataTypeStr=boolean
  Compare To Constant1 : simulink/Logic and Bit Operations/Compare To Constant  relop=>=  const=x_t_max_oper  OutDataTypeStr=boolean
  Compare To Constant2 : simulink/Logic and Bit Operations/Compare To Constant  relop=<=  const=x_t_min_emer  OutDataTypeStr=boolean
  Compare To Constant3 : simulink/Logic and Bit Operations/Compare To Constant  relop=>=  const=x_t_max_emer  OutDataTypeStr=boolean
  x_t_min_oper : Outport  OutDataTypeStr=boolean  PortDimensions=1  SampleTime=0
  x_t_max_oper : Outport  Port=2  OutDataTypeStr=boolean  PortDimensions=1  SampleTime=0
  x_t_min_emer : Outport  Port=3  OutDataTypeStr=boolean  PortDimensions=1  SampleTime=0
  x_t_max_emer : Outport  Port=4  OutDataTypeStr=boolean  PortDimensions=1  SampleTime=0
  wires:
  Compare To Constant2/1 -> x_t_min_emer/1
  Compare To Constant/1 -> x_t_min_oper/1
  Compare To Constant1/1 -> x_t_max_oper/1
  x_t/1 -> Compare To Constant3/1, Compare To Constant2/1, Compare To Constant1/1, Compare To Constant/1
  Compare To Constant3/1 -> x_t_max_emer/1

== system sistema_fisico/Traslación del carro/Fuerza del cable del carro ==
  note: Posición de tambor del carro
  note: Velocidad del tambor del carro
  note: Posición del carro
  note: Velocidad del carro
  note: Fuerza del cable del carro
  x_td : Inport
  x_t : Inport  Port=2
  x_td_dot : Inport  Port=3
  x_t_dot : Inport  Port=4
  Gain : Gain  Gain=K_tw
  Gain1 : Gain  Gain=b_tw
  Sum2 : Sum  Inputs=+-
  Sum3 : Sum  Inputs=+-
  Sum4 : Sum
  F_tw : Outport
  wires:
  x_td_dot/1 -> Sum3/1
  x_td/1 -> Sum2/1
  x_t_dot/1 -> Sum3/2
  x_t/1 -> Sum2/2
  Sum4/1 -> F_tw/1
  Gain/1 -> Sum4/1
  Sum2/1 -> Gain/1
  Gain1/1 -> Sum4/2
  Sum3/1 -> Gain1/1

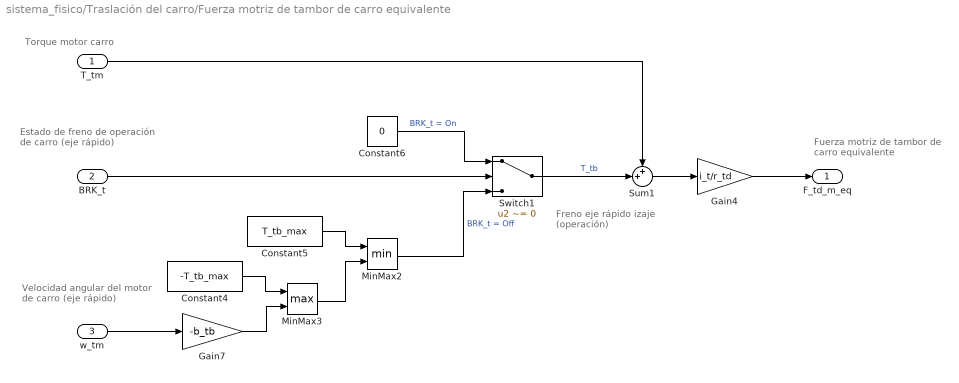
== system sistema_fisico/Traslación del carro/Fuerza motriz de tambor de carro equivalente ==
  note: Fuerza motriz de tambor
      | de carro equivalente
  note: Torque motor carro
  note: Freno eje rápido izaje
      | (operación)
  note: Estado de freno de
      | operación de carro
      | (eje rápido)
  note: Velocidad angular
      | del motor de carro
      | (eje rápido)
  T_tm : Inport
  BRK_t : Inport  Port=2  OutDataTypeStr=boolean
  w_tm : Inport  Port=3
  Constant4 : Constant  Value=-T_tb_max
  Constant5 : Constant  Value=T_tb_max
  Constant6 : Constant  Value=0
  Gain4 : Gain  Gain=i_t/r_td
  Gain7 : Gain  Gain=-b_tb
  MinMax2 : MinMax  Inputs=2
  MinMax3 : MinMax  Function=max  Inputs=2
  Sum1 : Sum  Inputs=++|
  Switch1 : Switch  Criteria=u2 ~= 0
  F_td_m_eq : Outport
  wires:
  MinMax3/1 -> MinMax2/2
  MinMax2/1 -> Switch1/3  "BRK_t = Off"
  Constant4/1 -> MinMax3/1
  T_tm/1 -> Sum1/1
  w_tm/1 -> Gain7/1
  Constant5/1 -> MinMax2/1
  Gain7/1 -> MinMax3/2
  BRK_t/1 -> Switch1/2
  Constant6/1 -> Switch1/1  "BRK_t = On"
  Sum1/1 -> Gain4/1
  Switch1/1 -> Sum1/2  "T_tb"
  Gain4/1 -> F_td_m_eq/1

== system sistema_fisico/Traslación del carro/Variables de estado derivadas ==
  note: Normalizar ángulo en
      | rango 0 a 2*pi
  note: Radio del tambor
  note: Caja reductora
      | entre motor y tambor
  note: Velocidad angular del motor del carro
  note: Velocidad de la carga sin balanceo
  note: Posición angular del motor del carro
  note: Caja reductora
      | entre motor y tambor
  note: Radio del tambor
  note: Posición horizontal
      | del tambor del carro
  x_td_dot : Inport
  x_td : Inport  Port=2
  Constant : Constant  Value=2*pi
  Gain1 : Gain  Gain=1/r_td
  Gain2 : Gain  Gain=1/r_td
  Gain3 : Gain  Gain=i_t
  Gain4 : Gain  Gain=i_t
  Mod1 : Math  Operator=mod  SaturateOnIntegerOverflow=on
  w_tm : Outport
  theta_tm : Outport  Port=2
  wires:
  Gain1/1 -> Gain3/1  "w_td"
  x_td_dot/1 -> Gain1/1
  Gain3/1 -> w_tm/1  "w_tm"
  x_td/1 -> Gain2/1
  Gain2/1 -> Gain4/1  "theta_td"
  Gain4/1 -> Mod1/1  "theta_tm_raw"
  Mod1/1 -> theta_tm/1
  Constant/1 -> Mod1/2

== system sistema_fisico/Carga suspendida/Parámetros de carga/Generate random load  ==
  note: Masa de contenedor
      | Condiciones nominales: M_c_min <= M_cx <= M_c_max
      | Condición de sobrecarga: M_cx > M_c_max
  note: Condición de sobrecarga
  note: Masa del contenedor y carga
  note: Se actualiza la masa del contenedor de carga
      | cuando se cierran los twistlocks (TL K ↑)
  Trigger : TriggerPort  VariantControl=Variant  PortDimensions=1
  Constant : Constant  Value=M_c_min
  Constant1 : Constant  Value=M_c_max
  Constant2 : Constant  Value=1.25 * M_c_max
  Constant4 : Constant  Value=M_c_max
  MATLAB Function : MATLAB Function  TreatAsAtomicUnit=on
  Switch1 : Switch  Criteria=u2 ~= 0
  Switch2 : Switch  Criteria=u2 ~= 0
  h_c5 : Constant  Value=overload
  M_cx : Outport  OutDataTypeStr=double  PortDimensions=1  InitialOutput=0
  wires:
  MATLAB Function/1(y) -> M_cx/1
  Constant/1 -> Switch1/3
  Constant1/1 -> Switch1/1
  Constant2/1 -> Switch2/1
  Constant4/1 -> Switch2/3
  h_c5/1 -> Switch1/2, Switch2/2
  Switch1/1 -> MATLAB Function/1(min)
  Switch2/1 -> MATLAB Function/2(max)

== matlab function sistema_fisico/Carga suspendida/Perfil de obstáculos/MATLAB Function ==
  data: x_l input; y_c0_x_l output; TLK input; H_c input; x_t_min_oper input; x_t_max_oper input; y_h_min_oper input; y_c0 output size=[1, 1651]
function [y_c0_x_l,y_c0] = update_perfil_obstactulos(x_l, TLK, H_c, x_t_min_oper, x_t_max_oper, y_h_min_oper)
    % Actualiza el perfil de obstaculos
    % Entradas:
    % 1) x_l: posición horizontal de la carga 
    % 2) TLK: twistlocks
    % 3) H_c: alto del container estándar
    % 4) x_t_min_oper: límite de operación mínimo de posición horizontal
    % del carro
    % 5) x_t_max_oper: límite de operación máximo de posición horizontal
    % del carro
    % 6) y_h_min_oper: límite de operación mínimo de posición vertical
    % de izaje
    % Salidas:
    % 1) y_c0_x_l: perfil de obstáculo para la posición x_l y tiempo actual
    % 2) y_c0: perfil de obstáculo (vector de altura de obstáculos en
    % función de posición horizontal) para el tiempo actual
    
    persistent y_c0_prev x;
    
    if isempty(y_c0_prev)
        % Inicializar y_c0_prev si es la primera ejecución
        x_min = x_t_min_oper - H_c/2;
        x_max = x_t_max_oper + H_c/2;
        x = x_min:0.05:x_max; % Vector de posiciones horizontales
        y_c0_prev = y_h_min_oper * ones(1, size(x,2)); %Inicializa y_c0_prev con la posición vertical mínima
    end
    
    % Buscar índices donde x está en el rango [x_l ± H_c/2]
    indices = find((x >= (x_l - H_c/2)) & (x <= (x_l + H_c/2)));
    
    % Actualizar y_c0 para dichas posiciones.
    y_c0 = y_c0_prev; % Empieza con valores previos
    
    if (TLK)  % Si se abren los twistlocks (se suelta el contenedor)
        y_c0(indices) = y_c0(indices) + H_c;
    else      % Si se cierran los twistlocks (se agarra el contenedor)
        y_c0(indices) = y_c0(indices) - H_c;
    end
    
    % Buscar índice para x más cercano a x_l
    [~, index] = min(abs(x - x_l));
    y_c0_x_l = y_c0(index); % Actualiza valor de y_c0(x_l)
    
    % Guardar los valores actuales como previos para próxima iteración
    y_c0_prev = y_c0;
end

== matlab function sistema_fisico/Carga suspendida/Parámetros de carga/Generate random load /MATLAB Function ==
  data: y output; min input; max input
function y = update_random(min, max)
    persistent r;
    if isempty(r)
        rng('shuffle'); % Shuffle the seed ONCE at the start
    end
    r = randi([min, max]); % Generate a new random integer on trigger
    y = r;
end
